simulink model "PID_Controller"  (R2017b)
settings: Solver=ode5  StartTime=0.0  StopTime=13.4374  FixedStep=0.02  RelTol=1e-3
settings Model: Creator=Admin  LastModifiedBy=DELL
settings CodeAppCC: StateflowObjectComments=on

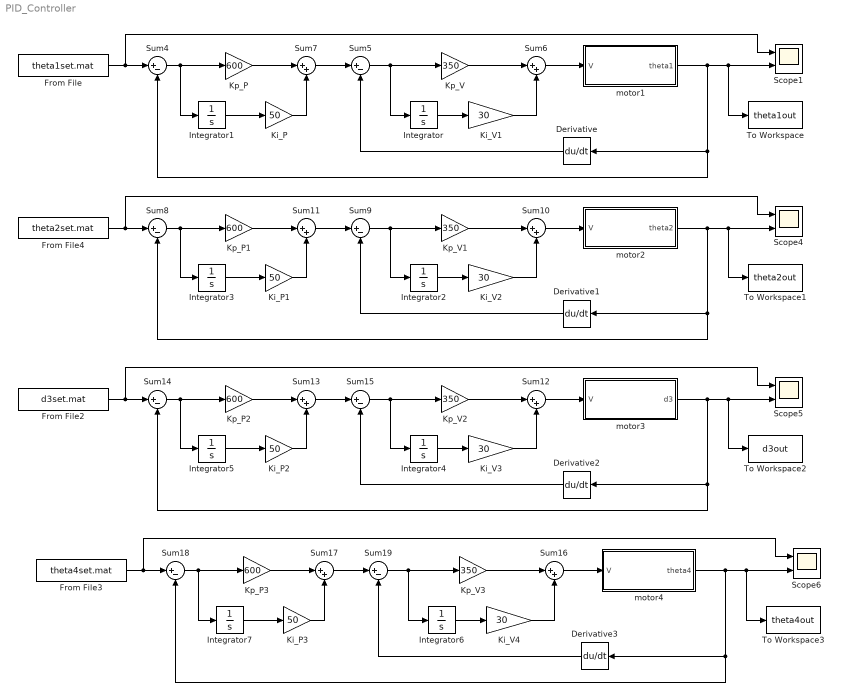
== system PID_Controller ==
  Derivative{,1..3} (4 alike) : Derivative
  From File : FromFile  FileName=theta1set.mat
  From File2 : FromFile  FileName=d3set.mat
  From File3 : FromFile  FileName=theta4set.mat
  From File4 : FromFile  FileName=theta2set.mat
  Integrator{,1..7} (8 alike) : Integrator
  Ki_P{,1..3} (4 alike) : Gain  Gain=50
  Ki_V{1..4} (4 alike) : Gain  Gain=30
  Kp_P{,1..3} (4 alike) : Gain  Gain=600
  Kp_V{,1..3} (4 alike) : Gain  Gain=350
  Scope{1,4..6} (4 alike) : Scope  NumInputPorts=2
  Sum{6..7,10..13,16..17} (8 alike) : Sum  Inputs=|++
  Sum{4..5,8..9,14..15,18..19} (8 alike) : Sum  Inputs=|+-
  To Workspace : ToWorkspace  VariableName=theta1out  SampleTime=-1
  To Workspace1 : ToWorkspace  VariableName=theta2out  SampleTime=-1
  To Workspace2 : ToWorkspace  VariableName=d3out  SampleTime=-1
  To Workspace3 : ToWorkspace  VariableName=theta4out  SampleTime=-1
  motor1 : Subsystem  mask{Ki=0.1, Kb=0.1, L=0.5, R=2, Jeff=0.02, Beff=0.2, N=100}
  motor2 : Subsystem  mask{Ki=0.1, Kb=0.1, L=0.5, R=2, Jeff=0.02, Beff=0.2, N=100}
  motor3 : Subsystem  mask{Ki=0.1, Kb=0.1, L=0.5, R=2, Jeff=0.02, Beff=0.2, N=100}
  motor4 : Subsystem  mask{Ki=0.1, Kb=0.1, L=0.5, R=2, Jeff=0.02, Beff=0.2, N=100}
  wires:
  Sum16/1 -> motor4/1(V)
  motor4/1(theta4) -> Sum18/2, Derivative3/1, To Workspace3/1, Scope6/2
  Kp_V3/1 -> Sum16/1
  Integrator6/1 -> Ki_V4/1
  Sum17/1 -> Sum19/1
  From File3/1 -> Scope6/1, Sum18/1
  Integrator7/1 -> Ki_P3/1
  Kp_P3/1 -> Sum17/1
  Derivative3/1 -> Sum19/2
  Ki_V4/1 -> Sum16/2
  Sum19/1 -> Integrator6/1, Kp_V3/1
  Ki_P3/1 -> Sum17/2
  Sum18/1 -> Integrator7/1, Kp_P3/1
  Sum10/1 -> motor2/1(V)
  motor2/1(theta2) -> Sum8/2, Derivative1/1, To Workspace1/1, Scope4/2
  Sum14/1 -> Integrator5/1, Kp_P2/1
  Kp_V2/1 -> Sum12/1
  Sum15/1 -> Integrator4/1, Kp_V2/1
  From File4/1 -> Scope4/1, Sum8/1
  Kp_P/1 -> Sum7/1
  Integrator/1 -> Ki_V1/1
  motor3/1(d3) -> Sum14/2, Derivative2/1, To Workspace2/1, Scope5/2
  Ki_P/1 -> Sum7/2
  Sum8/1 -> Integrator3/1, Kp_P1/1
  Ki_V3/1 -> Sum12/2
  Derivative1/1 -> Sum9/2
  Sum13/1 -> Sum15/1
  Ki_V2/1 -> Sum10/2
  Integrator1/1 -> Ki_P/1
  motor1/1(theta1) -> Sum4/2, Derivative/1, To Workspace/1, Scope1/2
  Derivative/1 -> Sum5/2
  Sum7/1 -> Sum5/1
  Ki_V1/1 -> Sum6/2
  Sum5/1 -> Integrator/1, Kp_V/1
  From File/1 -> Scope1/1, Sum4/1
  Kp_V1/1 -> Sum10/1
  Integrator3/1 -> Ki_P1/1
  Integrator2/1 -> Ki_V2/1
  Sum4/1 -> Integrator1/1, Kp_P/1
  Kp_P1/1 -> Sum11/1
  Ki_P1/1 -> Sum11/2
  Sum9/1 -> Integrator2/1, Kp_V1/1
  From File2/1 -> Scope5/1, Sum14/1
  Sum12/1 -> motor3/1(V)
  Derivative2/1 -> Sum15/2
  Kp_P2/1 -> Sum13/1
  Integrator5/1 -> Ki_P2/1
  Kp_V/1 -> Sum6/1
  Integrator4/1 -> Ki_V3/1
  Sum6/1 -> motor1/1(V)
  Ki_P2/1 -> Sum13/2
  Sum11/1 -> Sum9/1

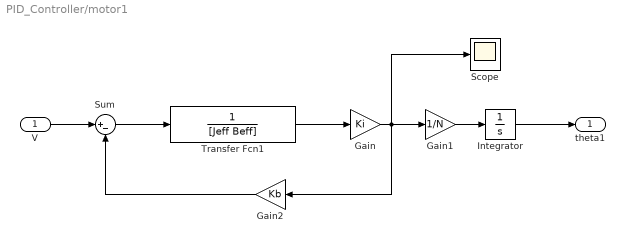
== system PID_Controller/motor1 ==
  V : Inport
  Gain : Gain  Gain=Ki
  Gain1 : Gain  Gain=1/N
  Gain2 : Gain  Gain=Kb
  Integrator : Integrator
  Scope : Scope
  Sum : Sum  Inputs=|+-
  Transfer Fcn1 : TransferFcn  Denominator=[Jeff Beff]
  theta1 : Outport
  wires:
  Transfer Fcn1/1 -> Gain/1
  Gain2/1 -> Sum/2
  V/1 -> Sum/1
  Sum/1 -> Transfer Fcn1/1
  Gain/1 -> Gain1/1, Gain2/1, Scope/1
  Gain1/1 -> Integrator/1
  Integrator/1 -> theta1/1

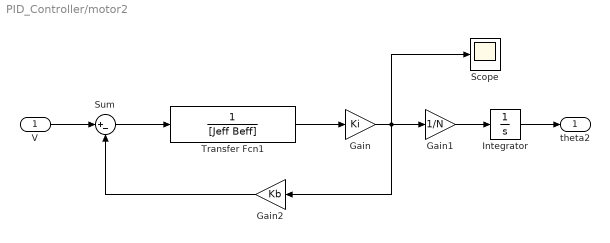
== system PID_Controller/motor2 ==
  V : Inport
  Gain : Gain  Gain=Ki
  Gain1 : Gain  Gain=1/N
  Gain2 : Gain  Gain=Kb
  Integrator : Integrator  InitialCondition=90
  Scope : Scope
  Sum : Sum  Inputs=|+-
  Transfer Fcn1 : TransferFcn  Denominator=[Jeff Beff]
  theta2 : Outport
  wires:
  Transfer Fcn1/1 -> Gain/1
  Gain1/1 -> Integrator/1
  Gain2/1 -> Sum/2
  V/1 -> Sum/1
  Sum/1 -> Transfer Fcn1/1
  Gain/1 -> Gain1/1, Gain2/1, Scope/1
  Integrator/1 -> theta2/1

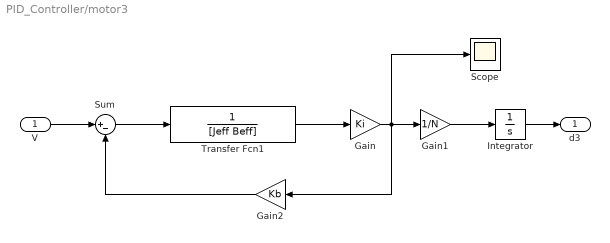
== system PID_Controller/motor3 ==
  V : Inport
  Gain : Gain  Gain=Ki
  Gain1 : Gain  Gain=1/N
  Gain2 : Gain  Gain=Kb
  Integrator : Integrator
  Scope : Scope
  Sum : Sum  Inputs=|+-
  Transfer Fcn1 : TransferFcn  Denominator=[Jeff Beff]
  d3 : Outport
  wires:
  Transfer Fcn1/1 -> Gain/1
  Gain1/1 -> Integrator/1
  Integrator/1 -> d3/1
  Gain2/1 -> Sum/2
  V/1 -> Sum/1
  Sum/1 -> Transfer Fcn1/1
  Gain/1 -> Gain1/1, Gain2/1, Scope/1

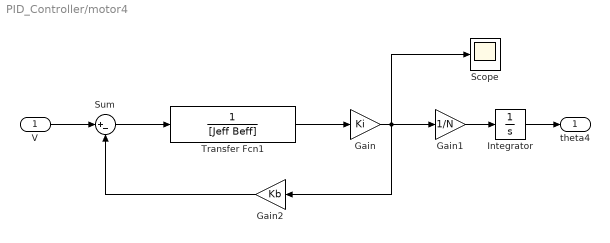
== system PID_Controller/motor4 ==
  V : Inport
  Gain : Gain  Gain=Ki
  Gain1 : Gain  Gain=1/N
  Gain2 : Gain  Gain=Kb
  Integrator : Integrator
  Scope : Scope
  Sum : Sum  Inputs=|+-
  Transfer Fcn1 : TransferFcn  Denominator=[Jeff Beff]
  theta4 : Outport
  wires:
  Transfer Fcn1/1 -> Gain/1
  Gain/1 -> Gain1/1, Gain2/1, Scope/1
  Gain1/1 -> Integrator/1
  Gain2/1 -> Sum/2
  V/1 -> Sum/1
  Sum/1 -> Transfer Fcn1/1
  Integrator/1 -> theta4/1
